simulink model "stm32f4_read_agm_imu_9a_target_demo"  (Simulink 7.3)
settings: Solver=ode3  SolverMode=SingleTasking  StartTime=0.0  StopTime=10.0  RelTol=1e-3
PreLoadFcn:
  | waijung.modelPreload; % Required for working with Waijung Blockset. Do not remove.
undefined symbols (not defined in the file): HSEOSC, Link, LQFP176, ST, STM32F417IG
libraries: simulink x21, stm32f4_i2c_lib x19, stm32f4_device_config_lib x1
CloseFcn:
  | waijung.modelClose; % Required for working with Waijung Blockset. Do not remove.
settings Model: Creator=Krisada  LastModifiedBy=Krisada
settings OptimizationCC: OptimizeModelRefInitCode=on  LifeSpan=1
settings HardwareCC: ProdEndianess=LittleEndian  ProdHWDeviceType=ARM Compatible->Cortex - M4  TargetEndianess=LittleEndian  TargetHWDeviceType=ARM Compatible->Cortex - M4
settings RTWCC: SystemTargetFile=stm32f4.tlc  GenerateMakefile=off  TemplateMakefile=ert_default_tmf  Description=STM32F4 Target  ProcessScript=stm32f4_make_rtw_hook
settings CodeAppCC: IgnoreCustomStorageClasses=off
settings STFCustomTargetCC: ModelReferenceCompliant=off  CombineOutputUpdateFcns=on  ERTCustomFileBanners=on  SupportContinuousTime=off  SupportNonInlinedSFcns=off  SystemTargetFile=stm32f4.tlc
settings ERTTargetCC: MultiwordLength=2048  ModelReferenceCompliant=off  ParMdlRefBuildCompliant=off  CompOptLevelCompliant=off  ERTFirstTimeCompliant=off  ModelStepFunctionPrototypeControlCompliant=off  CPPClassGenCompliant=off  InlinedParameterPlacement=NonHierarchical  ERTSrcFileBannerTemplate=stm32f4_code_template.cgt  ERTHdrFileBannerTemplate=stm32f4_code_template.cgt  ERTDataSrcFileTemplate=stm32f4_code_template.cgt  ERTDataHdrFileTemplate=stm32f4_code_template.cgt  ERTCustomFileTemplate=stm32f4_file_process.tlc

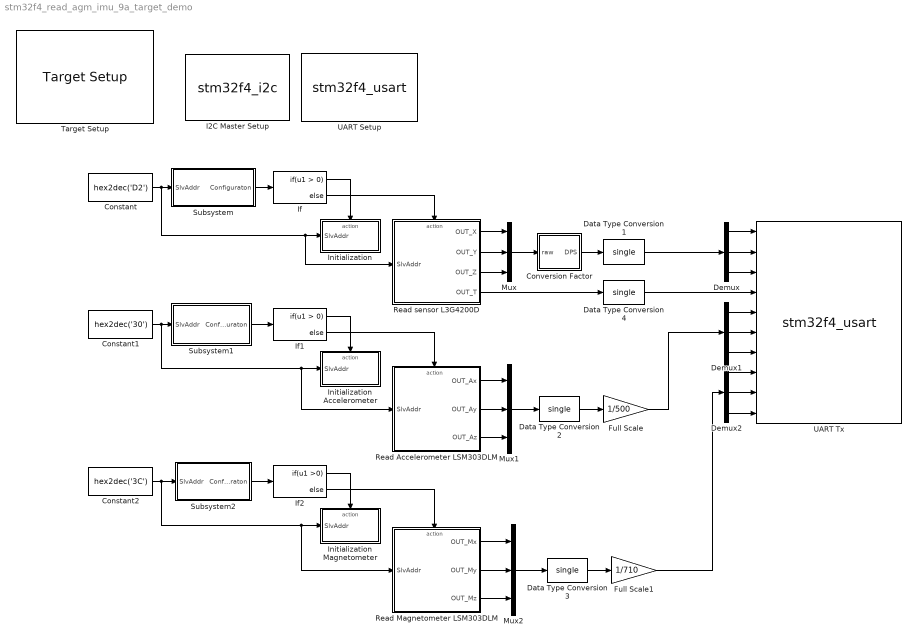
== system stm32f4_read_agm_imu_9a_target_demo ==
  Constant : Constant  Value=hex2dec('D2')  OutDataTypeMode=uint8  OutDataType=fixdt(1, 16)  OutScaling=2^0  OutDataTypeStr=uint8
  Constant1 : Constant  Value=hex2dec('30')  OutDataTypeMode=uint8  OutDataType=fixdt(1, 16)  OutScaling=2^0  OutDataTypeStr=uint8
  Constant2 : Constant  Value=hex2dec('3C')  OutDataTypeMode=uint8  OutDataType=fixdt(1, 16)  OutScaling=2^0  OutDataTypeStr=uint8
  Conversion Factor : Subsystem
  Data Type Conversion{1..4} (4 alike) : DataTypeConversion  OutDataTypeMode=single  OutDataType=fixdt(1, 16)  OutScaling=2^0  OutDataTypeStr=single
  Demux : Demux  Outputs=3
  Demux1 : Demux  Outputs=3
  Demux2 : Demux  Outputs=3
  Full Scale : Gain  Gain=1/500  ParameterDataType=fixdt(1, 16)  ParameterScaling=2^0  OutDataType=fixdt(1, 16)  OutScaling=2^0
  Full Scale1 : Gain  Gain=1/710  ParameterDataType=fixdt(1, 16)  ParameterScaling=2^0  OutDataType=fixdt(1, 16)  OutScaling=2^0
  I2C Master Setup : S-Function  FunctionName=stm32f4_i2c  Parameters=configuration,module,transfer,clkspeed,timeout,sdapin,sclpin,writecount,readcount,inputtypearray,outputtypearray,confstr,sampletime,sampletimestr,blockid  EnableBusSupport=off  mask(stm32f4_i2c){configuration=Setup, module=1, lastmodule=1, transfer=Blocking, dutycycle=TLow/THigh = 2, clkspeed=100, timeout=25, writecount=0, readcount=0, sdapin=B7, sclpin=B6, waitwritetime=0, inputtypearray=[0], outputtypearray=[0], confstr=["B","7","B","6","1","1","6","0","I2C_DutyCycle_2","0","off"], sampletime=-1, sampletimestr=0.01, blockid=I2CMasterSetup}
      mask prompts: module "I2C Module"; lastmodule "Last module"; transfer "Transfer mode"; dutycycle "Duty cycle in fast mode"; clkspeed "Clock speed (kHz)"; timeout "Timeout (ms)"; writecount "Bytes write count"; readcount "Bytes read count"; sdapin "SDA pin"; sclpin "SCL pin"; waitwritetime "Wait write time (ms), default is 0"; inputtypearray "Input type array"; outputtypearray "Output type array"; confstr "Configuration string"; sampletime "Sample time (sec)"; sampletimestr "Compiled sample time (sec) in string"
      mask init:
      | stm32f4_i2c_callback('init');
      mask Help: web(fullfile(waijungdocroot,'stm32f4_i2c_setup.htm'), '-browser')
      mask StyleString: popup(Setup|Transaction),popup(1|2|3),edit,popup(Blocking|Non-blocking),popup(TLow/THigh = 16/9|TLow/THigh = 2),edit,edit,edit,edit,popup(Not used|B7|B9),popup(Not used|B6|B8),edit,edit,edit,edit,edit,edit,edit
      mask CallbackString: stm32f4_i2c_callback('configuration');|stm32f4_i2c_callback('module');|||stm32f4_i2c_callback('dutycycle');|||stm32f4_i2c_callback('writecount');|stm32f4_i2c_callback('readcount');|stm32f4_i2c_callback('sdapin');|stm32f4_i2c_callback('sclpin');||||stm32f4_i2c_callback('confstr');|stm32f4_i2c_callback('sampletime');|stm32f4_i2c_callback('sampletimestr');|stm32f4_i2c_callback('blockid');
      mask Display: text(0.5, 0.5, 'Module: I2C1\nClock: 100kHz\nSDA/SCL Pin: B7/B6','ver','middle','hor','center');
  If : If
  If1 : If
  If2 : If  IfExpression=u1 >0
  Initialization : Subsystem
  Initialization Accelerometer : Subsystem
  Initialization Magnetometer : Subsystem
  Mux : Mux  Inputs=3
  Mux1 : Mux  Inputs=3
  Mux2 : Mux  Inputs=3
  Read Accelerometer LSM303DLM : Subsystem  TreatAsAtomicUnit=on
  Read Magnetometer LSM303DLM : Subsystem  TreatAsAtomicUnit=on
  Read sensor L3G4200D : Subsystem  TreatAsAtomicUnit=on
  Subsystem : Subsystem
  Subsystem1 : Subsystem
  Subsystem2 : Subsystem
  Target Setup : stm32f4_device_config_lib/Target Setup  Priority=100  compiler=GNU ARM  previous_compiler=GNU ARM  mcu=STM32F417IG (LQFP176)  mcustr=STM32F417IG  clockconfig=HSEOSC-8MHz  system_stm32f4xx_c_path=F:\trunk\targets\stm32f4_target\stm32f4\utils\system_stm32f4xx_default\STM32F40_41xxx\hseosc8mhz  showmemoryconfiguration=off  stacksize=0x2000  heapsize=0x2000  enableautocompiledownload=on  fullchiperase=off  programmerinterface=ST-Link  editctrlstr=on  compilercontrolstr=$(patsubst %, -I%, .) -mcpu=cortex-m4 -mthumb -mthumb-interwork -mfloat-abi=hard -mfpu=fpv4-sp-d16 -ffast-math -Wall -Wextra -Ofast  assemblercontrolstr=$(patsubst %, -I%, .) -mcpu=cortex-m4 -mthumb -mthumb-interwork -mfloat-abi=hard -mfpu=fpv4-sp-d16 -ffast-math -Wall -Wextra -Ofast -Wa,-amhls=$(<:.s=.lst) -D__STACK_SIZE=$(STACK_SIZE) -D__HEAP_SIZE=$(HEAP_SIZE)  linkercontrolstr=-T$(LD_SCRIPT) -g -Wl,-Map=$(MAP),--cref,--no-warn-mismatch -mcpu=cortex-m4 -mthumb -mthumb-interwork -mfloat-abi=hard -mfpu=fpv4-sp-d16 -specs=nosys.specs  runafterdownload=on  execprofile=None  profileruart=3  profilerbaud=500000  profilertxpin=D8  profilerinitstr=0.01,168000000,1680000,500000,0  manualsetsampletime=off  sampletime=0.01  blockid=TargetSetup  systickreloadvalue=1680000  hseval=8000000  lastprofileruart=3  hclk=168000000  flashorigin=0x8000000  flashlength=1024k  ramorigin=0x20000000  ramlength=128k  useextram=off
  UART Setup : S-Function  Priority=1  FunctionName=stm32f4_usart  Parameters=configuration,uartmodule,transfer,baudrate,inputtype,outputtype,confstr,binheaderarray,binterminatorarray,asciiheader,asciiterminator,bindatalength,packetmode,varname,sampletime,sampletimestr,blockid  EnableBusSupport=off  mask(stm32f4_usart){configuration=Setup, uartmodule=3, baudrate=115200, databits=8, parity=No, stopbit=1, remaptxpin=D8, remaprxpin=Not used, flowcontrol=None, remapctspin=Not used, remaprtspin=Not used, advanceoptions=off, rxbuffersize=512, txbuffersize=512, transfer=Blocking, packetmode=Ascii, binheader='7E 7E', binterminator='03 03', porttype_double=1, porttype_single=0, porttype_int8=1, porttype_uint8=0, porttype_int16=0, porttype_uint16=0, porttype_int32=0, porttype_uint32=0, asciiformat='%d,%f', rx_asciiterminator=CRLF (0x0D 0x0A - "\r\n"), tx_asciiterminator=CR (0x0D - "\r"), storagename=<empty>, varname=, inputtype=[0], outputtype=[0], binheaderarray=[0], binterminatorarray=[0], bindatalength=0, asciiheader='', asciiterminator=[0], sampletime=-1, sampletimestr=0.01, blockid=UARTSetup, confstr=[ "dummy", "1", "D", "8", "0", "*", "*", "0", "*", "*", "0", "*", "*", "1", "4", "3", "1", "4", "1", "512", "512", "1", "3", "115200", "8", "No", "1", "None", "USART3"], lastmodule=3}
      mask prompts: uartmodule "UART Module"; baudrate "Baud rate (bps)"; databits "Data bits"; stopbit "Stop bit"; remaptxpin "Tx Pin"; remaprxpin "Rx Pin"; flowcontrol "Hardware flow control"; remapctspin "HW Flow control, CTS Pin"; remaprtspin "HW Flow control, RTS Pin"; advanceoptions "Advance options"; rxbuffersize "Rx buffer size (bytes)"; txbuffersize "Tx buffer size (bytes)"; packetmode "Packet mode"; binheader "Binary header (example: '7E 7E')"; binterminator "Binary terminator (example: '03 03')"; porttype_double "Number of data port, type DOUBLE"; porttype_single "Number of data port, type SINGLE"; porttype_int8 "Number of data port, type INT8"; porttype_uint8 "Number of data port, type UINT8"; porttype_int16 "Number of data port, type INT16"; porttype_uint16 "Number of data port, type UINT16"; porttype_int32 "Number of data port, type INT32"; porttype_uint32 "Number of data port, type UINT32"; asciiformat "Ascii format"; rx_asciiterminator "End of packet"; tx_asciiterminator "End of packet"; storagename "Buffer"; varname "Var name"; inputtype "Input data type"; outputtype "Output data type"; binheaderarray "Binary header"; binterminatorarray "Binary terminator"; bindatalength "Binary data length"; asciiheader "Ascii header (printf format)"; asciiterminator "Ascii terminator"; sampletime "Sample time (sec)"; sampletimestr "Compiled sample time (sec) in string"; confstr "Configuration string"; lastmodule "Last module selected"
      mask help:
      | Default STM32F4DISCOVERY + aMG F4 Connect 2 + aMG USB Converter N2 settings use
      |
      | USART3, Tx D8, Rx D9 and USB Serial Converter A.
      mask init:
      | stm32f4_usart_callback('init');
      mask Help: web(fullfile(waijungdocroot,'stm32f4_usart_setup.htm'), '-browser')
      mask StyleString: popup(Setup|Tx|Rx),popup(1|2|3|4|5|6),edit,popup(8),popup(No|Odd|Even),popup(0.5|1|1.5|2),popup(Not used|B10|C10|D8),popup(Not used|B11|C11|D9),popup(None|RTS|CTS|RTS/CTS),popup(Not used|B13|D11),popup(Not used|B14|D12),checkbox,popup(16|32|64|128|256|512|1024|2048),popup(16|32|64|128|256|512|1024|2048),popup(Blocking|Non-Blocking),popup(Ascii|Binary|String Buffer),edit,edit,edit,edit,edit,edit,edit,edit,edit,edit,edit,popup(CR (0x0D - "\r")|LF (0x0A - "\n")|CRLF (0x0D 0x0A - "\r\n")),popup(CR (0x0D - "\r")|LF (0x0A - "\n")|CRLF (0x0D 0x0A - "\r\n")|None),popup(<empty>),edit,edit,edit,edit,edit,edit,edit,edit,edit,edit,edit,edit,edit
      mask CallbackString: stm32f4_usart_callback('configuration');|stm32f4_usart_callback('uartmodule');|stm32f4_usart_callback('baudrate');||||||stm32f4_usart_callback('flowcontrol');|||stm32f4_usart_callback('advanceoptions');|||stm32f4_usart_callback('transfer');|stm32f4_usart_callback('packetmode');|stm32f4_usart_callback('binheader');|stm32f4_usart_callback('binterminator');|stm32f4_usart_callback('porttype');|stm32f4_usart_callback('porttype');|stm32f4_usart_callback('porttype');|stm32f4_usart_callback('porttype');|stm32f4_usart_callback('porttype');|stm32f4_usart_callback('porttype');|stm32f4_usart_callback('porttype');|stm32f4_usart_callback('porttype');|stm32f4_usart_callback('asciiformat');|stm32f4_usart_callback('rx_asciiterminator');|stm32f4_usart_callback('tx_asciiterminator');|stm32f4_usart_callback('storagename');|stm32f4_usart_callback('varname');||||||||stm32f4_usart_callback('sampletime');|stm32f4_usart_callback('sampletimestr');|stm32f4_usart_callback('blockid');||
      mask Display: text(0.5, 0.5, 'Module: USART3_Setup\nBaud (Bps): 115200\nDMA Buffer: 512/-\nTx/Rx Pin: D8/-','ver','middle','hor','center');
  UART Tx : S-Function  Priority=1  FunctionName=stm32f4_usart  Parameters=configuration,uartmodule,transfer,baudrate,inputtype,outputtype,confstr,binheaderarray,binterminatorarray,asciiheader,asciiterminator,bindatalength,packetmode,varname,sampletime,sampletimestr,blockid  EnableBusSupport=off  mask(stm32f4_usart){configuration=Tx, uartmodule=3, baudrate=115200, databits=8, parity=No, stopbit=1, remaptxpin=Not used, remaprxpin=Not used, flowcontrol=None, remapctspin=Not used, remaprtspin=Not used, advanceoptions=off, rxbuffersize=512, txbuffersize=512, transfer=Blocking, packetmode=Binary, binheader='7E 7E', binterminator='03 03', porttype_double=0, porttype_single=10, porttype_int8=0, porttype_uint8=0, porttype_int16=0, porttype_uint16=0, porttype_int32=0, porttype_uint32=0, asciiformat='value=%d,%f', rx_asciiterminator=CRLF (0x0D 0x0A - "\r\n"), tx_asciiterminator=CRLF (0x0D 0x0A - "\r\n"), storagename=<empty>, varname=, inputtype=[10  1 1 1 1 1 1 1 1 1 1], outputtype=[0], binheaderarray=[2 126  126], binterminatorarray=[2 3  3], bindatalength=40, asciiheader='value=%d,%f\r\n', asciiterminator=[2 13 10], sampletime=-1, sampletimestr=0.01, blockid=UARTTx, confstr=[ "dummy", "0", "*", "*", "0", "*", "*", "0", "*", "*", "0", "*", "*", "1", "4", "3", "1", "4", "1", "512", "512", "1", "3", "115200", "8", "No", "1", "None", "USART3"], lastmodule=1}
      mask prompts: uartmodule "UART Module"; baudrate "Baud rate (bps)"; databits "Data bits"; stopbit "Stop bit"; remaptxpin "Tx Pin"; remaprxpin "Rx Pin"; flowcontrol "Hardware flow control"; remapctspin "HW Flow control, CTS Pin"; remaprtspin "HW Flow control, RTS Pin"; advanceoptions "Advance options"; rxbuffersize "Rx buffer size (bytes)"; txbuffersize "Tx buffer size (bytes)"; packetmode "Packet mode"; binheader "Binary header (example: '7E 7E')"; binterminator "Binary terminator (example: '03 03')"; porttype_double "Number of data port, type DOUBLE"; porttype_single "Number of data port, type SINGLE"; porttype_int8 "Number of data port, type INT8"; porttype_uint8 "Number of data port, type UINT8"; porttype_int16 "Number of data port, type INT16"; porttype_uint16 "Number of data port, type UINT16"; porttype_int32 "Number of data port, type INT32"; porttype_uint32 "Number of data port, type UINT32"; asciiformat "Ascii format"; rx_asciiterminator "End of packet"; tx_asciiterminator "End of packet"; storagename "Buffer"; varname "Var name"; inputtype "Input data type"; outputtype "Output data type"; binheaderarray "Binary header"; binterminatorarray "Binary terminator"; bindatalength "Binary data length"; asciiheader "Ascii header (printf format)"; asciiterminator "Ascii terminator"; sampletime "Sample time (sec)"; sampletimestr "Compiled sample time (sec) in string"; confstr "Configuration string"; lastmodule "Last module selected"
      mask help:
      | Data type for Ascii format
      | %u, %i, %d, %o, %x: uint32
      | %e, %g, %f: single
      | %c: int8
      mask init:
      | stm32f4_usart_callback('init');
      mask Help: web(fullfile(waijungdocroot,'stm32f4_usart_tx.htm'), '-browser')
      mask StyleString: popup(Setup|Tx|Rx),popup(1|2|3|4|5|6),edit,popup(8),popup(No|Odd|Even),popup(0.5|1|1.5|2),popup(Not used|A9|B6),popup(Not used|A10|B7),popup(None|RTS|CTS|RTS/CTS),popup(Not used|A11),popup(Not used|A12),checkbox,popup(16|32|64|128|256|512|1024|2048),popup(16|32|64|128|256|512|1024|2048),popup(Blocking|Non-Blocking),popup(Ascii|Binary|String Buffer),edit,edit,edit,edit,edit,edit,edit,edit,edit,edit,edit,popup(CR (0x0D - "\r")|LF (0x0A - "\n")|CRLF (0x0D 0x0A - "\r\n")),popup(CR (0x0D - "\r")|LF (0x0A - "\n")|CRLF (0x0D 0x0A - "\r\n")|None),popup(<empty>),edit,edit,edit,edit,edit,edit,edit,edit,edit,edit,edit,edit,edit
      mask CallbackString: stm32f4_usart_callback('configuration');|stm32f4_usart_callback('uartmodule');|stm32f4_usart_callback('baudrate');||||||stm32f4_usart_callback('flowcontrol');|||stm32f4_usart_callback('advanceoptions');|||stm32f4_usart_callback('transfer');|stm32f4_usart_callback('packetmode');|stm32f4_usart_callback('binheader');|stm32f4_usart_callback('binterminator');|stm32f4_usart_callback('porttype');|stm32f4_usart_callback('porttype');|stm32f4_usart_callback('porttype');|stm32f4_usart_callback('porttype');|stm32f4_usart_callback('porttype');|stm32f4_usart_callback('porttype');|stm32f4_usart_callback('porttype');|stm32f4_usart_callback('porttype');|stm32f4_usart_callback('asciiformat');|stm32f4_usart_callback('rx_asciiterminator');|stm32f4_usart_callback('tx_asciiterminator');|stm32f4_usart_callback('storagename');|stm32f4_usart_callback('varname');||||||||stm32f4_usart_callback('sampletime');|stm32f4_usart_callback('sampletimestr');|stm32f4_usart_callback('blockid');||
      mask Display: text(0.95, 0.5, 'Module: USART3_Tx\nPacket: Binary\nTransfer: Blocking\nTs (sec): 0.01','ver','middle','hor','right'); port_label('input', 1,'single'); port_label('input', 2,'single'); port_label('input', 3,'single'); port_label('input', 4,'single'); port_label('input', 5,'single'); port_label('input', 6,'single'); port_label('input', 7,'single'); port_label('input', 8,'single'); port_label('input', 9,'single'); port_label('input', 10,'single');
  wires:
  Subsystem/1(Configuraton) -> If/1
  Read sensor L3G4200D/1(OUT_X) -> Mux/1
  Read sensor L3G4200D/2(OUT_Y) -> Mux/2
  Read sensor L3G4200D/3(OUT_Z) -> Mux/3
  Conversion Factor/1(DPS) -> Data Type Conversion1/1
  Mux/1 -> Conversion Factor/1(raw)
  Data Type Conversion1/1 -> Demux/1
  If/1 -> Initialization/Action
  If/2 -> Read sensor L3G4200D/Action
  Subsystem1/1(Configuraton) -> If1/1
  Read Accelerometer LSM303DLM/1(OUT_Ax) -> Mux1/1
  Data Type Conversion2/1 -> Full Scale/1
  If1/1 -> Initialization Accelerometer/Action
  If1/2 -> Read Accelerometer LSM303DLM/Action
  Read Accelerometer LSM303DLM/2(OUT_Ay) -> Mux1/2
  Read Accelerometer LSM303DLM/3(OUT_Az) -> Mux1/3
  Mux1/1 -> Data Type Conversion2/1
  Full Scale/1 -> Demux1/1
  Read Magnetometer LSM303DLM/1(OUT_Mx) -> Mux2/1
  Data Type Conversion3/1 -> Full Scale1/1
  If2/1 -> Initialization Magnetometer/Action
  If2/2 -> Read Magnetometer LSM303DLM/Action
  Read Magnetometer LSM303DLM/2(OUT_My) -> Mux2/2
  Read Magnetometer LSM303DLM/3(OUT_Mz) -> Mux2/3
  Mux2/1 -> Data Type Conversion3/1
  Full Scale1/1 -> Demux2/1
  Subsystem2/1(Configuraton) -> If2/1
  Constant/1 -> Subsystem/1(SlvAddr), Initialization/1(SlvAddr), Read sensor L3G4200D/1(SlvAddr)
  Constant1/1 -> Subsystem1/1(SlvAddr), Initialization Accelerometer/1(SlvAddr), Read Accelerometer LSM303DLM/1(SlvAddr)
  Constant2/1 -> Subsystem2/1(SlvAddr), Initialization Magnetometer/1(SlvAddr), Read Magnetometer LSM303DLM/1(SlvAddr)
  Read sensor L3G4200D/4(OUT_T) -> Data Type Conversion4/1
  Demux/1 -> UART Tx/1
  Demux/2 -> UART Tx/2
  Demux/3 -> UART Tx/3
  Demux1/1 -> UART Tx/5
  Demux1/2 -> UART Tx/6
  Demux1/3 -> UART Tx/7
  Demux2/1 -> UART Tx/8
  Demux2/2 -> UART Tx/9
  Demux2/3 -> UART Tx/10
  Data Type Conversion4/1 -> UART Tx/4

== system stm32f4_read_agm_imu_9a_target_demo/Conversion Factor ==
  raw : Inport
  Constant : Constant  Value=2^15  OutDataType=fixdt(1, 16)  OutScaling=2^0
  Divide : Product  Inputs=*/  OutDataType=fixdt(1, 16)  OutScaling=2^-10
  Full Scale : Gain  Gain=250  ParameterDataType=fixdt(1, 16)  ParameterScaling=2^0  OutDataType=fixdt(1, 16)  OutScaling=2^0
  DPS : Outport
  wires:
  Constant/1 -> Divide/2
  Divide/1 -> Full Scale/1
  raw/1 -> Divide/1
  Full Scale/1 -> DPS/1

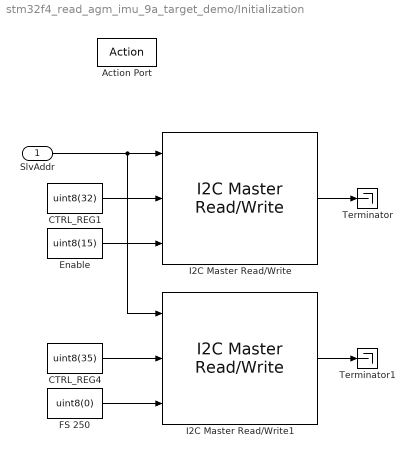
== system stm32f4_read_agm_imu_9a_target_demo/Initialization ==
  SlvAddr : Inport  OutDataType=fixdt(1, 16)  OutScaling=2^0
  Action Port : ActionPort  ActionType=then
  CTRL_REG1 : Constant  Value=uint8(32)  OutDataType=fixdt(1, 16)  OutScaling=2^0
  CTRL_REG4 : Constant  Value=uint8(35)  OutDataType=fixdt(1, 16)  OutScaling=2^0
  Enable : Constant  Value=uint8(15)  OutDataType=fixdt(1, 16)  OutScaling=2^0
  FS 250 : Constant  Value=uint8(0)  OutDataType=fixdt(1, 16)  OutScaling=2^0
  I2C Master Read/Write : stm32f4_i2c_lib/I2C Master Read//Write  configuration=Transaction  module=1  lastmodule=3  transfer=Blocking  dutycycle=TLow/THigh = 2  clkspeed=400  timeout=25  writecount=2  readcount=0  sdapin=C9  sclpin=A8  waitwritetime=0  forcestop=off  inputtypearray=[3 3 3 3]  outputtypearray=[1 3]  confstr="[\"C\",\"9\",\"A\",\"8\",\"1\",\"1\",\"6\",\"0\",\"I2C_DutyCycle_2\",\"0\",\"off\"]"  sampletime=-1  sampletimestr=0.01  blockid=InitializationI2CMasterReadWrite
  I2C Master Read/Write1 : stm32f4_i2c_lib/I2C Master Read//Write  configuration=Transaction  module=1  lastmodule=3  transfer=Blocking  dutycycle=TLow/THigh = 2  clkspeed=400  timeout=25  writecount=2  readcount=0  sdapin=C9  sclpin=A8  waitwritetime=0  forcestop=off  inputtypearray=[3 3 3 3]  outputtypearray=[1 3]  confstr="[\"C\",\"9\",\"A\",\"8\",\"1\",\"1\",\"6\",\"0\",\"I2C_DutyCycle_2\",\"0\",\"off\"]"  sampletime=-1  sampletimestr=0.01  blockid=InitializationI2CMasterReadWrite1
  Terminator : Terminator
  Terminator1 : Terminator
  wires:
  CTRL_REG1/1 -> I2C Master Read/Write/2
  Enable/1 -> I2C Master Read/Write/3
  CTRL_REG4/1 -> I2C Master Read/Write1/2
  FS 250/1 -> I2C Master Read/Write1/3
  SlvAddr/1 -> I2C Master Read/Write/1, I2C Master Read/Write1/1
  I2C Master Read/Write/1 -> Terminator/1
  I2C Master Read/Write1/1 -> Terminator1/1

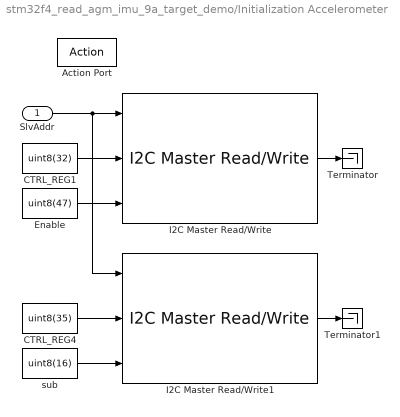
== system stm32f4_read_agm_imu_9a_target_demo/Initialization Accelerometer ==
  SlvAddr : Inport  OutDataType=fixdt(1, 16)  OutScaling=2^0
  Action Port : ActionPort  ActionType=then
  CTRL_REG1 : Constant  Value=uint8(32)  OutDataType=fixdt(1, 16)  OutScaling=2^0
  CTRL_REG4 : Constant  Value=uint8(35)  OutDataType=fixdt(1, 16)  OutScaling=2^0
  Enable : Constant  Value=uint8(47)  OutDataType=fixdt(1, 16)  OutScaling=2^0
  I2C Master Read/Write : stm32f4_i2c_lib/I2C Master Read//Write  configuration=Transaction  module=1  lastmodule=3  transfer=Blocking  dutycycle=TLow/THigh = 2  clkspeed=400  timeout=25  writecount=2  readcount=0  sdapin=C9  sclpin=A8  waitwritetime=0  forcestop=off  inputtypearray=[3 3 3 3]  outputtypearray=[1 3]  confstr="[\"C\",\"9\",\"A\",\"8\",\"1\",\"1\",\"6\",\"0\",\"I2C_DutyCycle_2\",\"0\",\"off\"]"  sampletime=-1  sampletimestr=0.01  blockid=InitializationAccelerometerI2CMasterReadWrite
  I2C Master Read/Write1 : stm32f4_i2c_lib/I2C Master Read//Write  configuration=Transaction  module=1  lastmodule=3  transfer=Blocking  dutycycle=TLow/THigh = 2  clkspeed=400  timeout=25  writecount=2  readcount=0  sdapin=C9  sclpin=A8  waitwritetime=0  forcestop=off  inputtypearray=[3 3 3 3]  outputtypearray=[1 3]  confstr="[\"C\",\"9\",\"A\",\"8\",\"1\",\"1\",\"6\",\"0\",\"I2C_DutyCycle_2\",\"0\",\"off\"]"  sampletime=-1  sampletimestr=0.01  blockid=InitializationAccelerometerI2CMasterReadWrite1
  Terminator : Terminator
  Terminator1 : Terminator
  sub : Constant  Value=uint8(16)  OutDataType=fixdt(1, 16)  OutScaling=2^0
  wires:
  Enable/1 -> I2C Master Read/Write/3
  CTRL_REG1/1 -> I2C Master Read/Write/2
  sub/1 -> I2C Master Read/Write1/3
  CTRL_REG4/1 -> I2C Master Read/Write1/2
  SlvAddr/1 -> I2C Master Read/Write/1, I2C Master Read/Write1/1
  I2C Master Read/Write/1 -> Terminator/1
  I2C Master Read/Write1/1 -> Terminator1/1

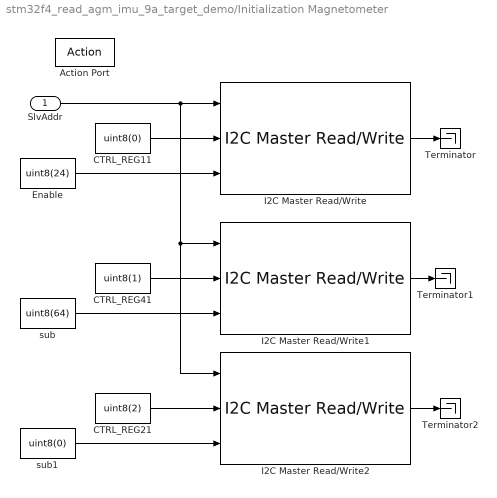
== system stm32f4_read_agm_imu_9a_target_demo/Initialization Magnetometer ==
  SlvAddr : Inport  OutDataType=fixdt(1, 16)  OutScaling=2^0
  Action Port : ActionPort  ActionType=then
  CTRL_REG11 : Constant  Value=uint8(0)  OutDataType=fixdt(1, 16)  OutScaling=2^0
  CTRL_REG21 : Constant  Value=uint8(2)  OutDataType=fixdt(1, 16)  OutScaling=2^0
  CTRL_REG41 : Constant  Value=uint8(1)  OutDataType=fixdt(1, 16)  OutScaling=2^0
  Enable : Constant  Value=uint8(24)  OutDataType=fixdt(1, 16)  OutScaling=2^0
  I2C Master Read/Write : stm32f4_i2c_lib/I2C Master Read//Write  configuration=Transaction  module=1  lastmodule=3  transfer=Blocking  dutycycle=TLow/THigh = 2  clkspeed=400  timeout=25  writecount=2  readcount=0  sdapin=C9  sclpin=A8  waitwritetime=0  forcestop=off  inputtypearray=[3 3 3 3]  outputtypearray=[1 3]  confstr="[\"C\",\"9\",\"A\",\"8\",\"1\",\"1\",\"6\",\"0\",\"I2C_DutyCycle_2\",\"0\",\"off\"]"  sampletime=-1  sampletimestr=0.01  blockid=InitializationMagnetometerI2CMasterReadWrite
  I2C Master Read/Write1 : stm32f4_i2c_lib/I2C Master Read//Write  configuration=Transaction  module=1  lastmodule=3  transfer=Blocking  dutycycle=TLow/THigh = 2  clkspeed=400  timeout=25  writecount=2  readcount=0  sdapin=C9  sclpin=A8  waitwritetime=0  forcestop=off  inputtypearray=[3 3 3 3]  outputtypearray=[1 3]  confstr="[\"C\",\"9\",\"A\",\"8\",\"1\",\"1\",\"6\",\"0\",\"I2C_DutyCycle_2\",\"0\",\"off\"]"  sampletime=-1  sampletimestr=0.01  blockid=InitializationMagnetometerI2CMasterReadWrite1
  I2C Master Read/Write2 : stm32f4_i2c_lib/I2C Master Read//Write  configuration=Transaction  module=1  lastmodule=3  transfer=Blocking  dutycycle=TLow/THigh = 2  clkspeed=400  timeout=25  writecount=2  readcount=0  sdapin=C9  sclpin=A8  waitwritetime=0  forcestop=off  inputtypearray=[3 3 3 3]  outputtypearray=[1 3]  confstr="[\"C\",\"9\",\"A\",\"8\",\"1\",\"1\",\"6\",\"0\",\"I2C_DutyCycle_2\",\"0\",\"off\"]"  sampletime=-1  sampletimestr=0.01  blockid=InitializationMagnetometerI2CMasterReadWrite2
  Terminator : Terminator
  Terminator1 : Terminator
  Terminator2 : Terminator
  sub : Constant  Value=uint8(64)  OutDataType=fixdt(1, 16)  OutScaling=2^0
  sub1 : Constant  Value=uint8(0)  OutDataType=fixdt(1, 16)  OutScaling=2^0
  wires:
  CTRL_REG11/1 -> I2C Master Read/Write/2
  Enable/1 -> I2C Master Read/Write/3
  CTRL_REG41/1 -> I2C Master Read/Write1/2
  sub/1 -> I2C Master Read/Write1/3
  I2C Master Read/Write/1 -> Terminator/1
  SlvAddr/1 -> I2C Master Read/Write/1, I2C Master Read/Write1/1, I2C Master Read/Write2/1
  sub1/1 -> I2C Master Read/Write2/3
  CTRL_REG21/1 -> I2C Master Read/Write2/2
  I2C Master Read/Write1/1 -> Terminator1/1
  I2C Master Read/Write2/1 -> Terminator2/1

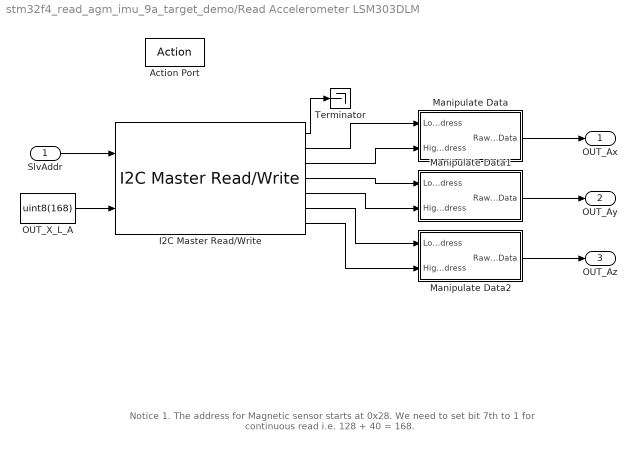
== system stm32f4_read_agm_imu_9a_target_demo/Read Accelerometer LSM303DLM ==
  note: Notice
      | 1. The address for Magnetic sensor starts at 0x28. We need to set bit 7th to 1 for continuous read i.e. 128 + 40 = 168.
  SlvAddr : Inport  OutDataType=fixdt(1, 16)  OutScaling=2^0
  Action Port : ActionPort  ActionType=else
  I2C Master Read/Write : stm32f4_i2c_lib/I2C Master Read//Write  configuration=Transaction  module=1  lastmodule=3  transfer=Blocking  dutycycle=TLow/THigh = 2  clkspeed=400  timeout=25  writecount=1  readcount=6  sdapin=C9  sclpin=A8  waitwritetime=0  forcestop=off  inputtypearray=[2 3 3]  outputtypearray=[7 3 3 3 3 3 3 3]  confstr="[\"C\",\"9\",\"A\",\"8\",\"1\",\"1\",\"6\",\"0\",\"I2C_DutyCycle_2\",\"0\",\"off\"]"  sampletime=-1  sampletimestr=0.01  blockid=ReadAccelerometerLSM303DLMI2CMasterReadWrite
  Manipulate Data : Subsystem
  Manipulate Data1 : Subsystem
  Manipulate Data2 : Subsystem
  OUT_X_L_A : Constant  Value=uint8(168)  OutDataType=fixdt(1, 16)  OutScaling=2^0
  Terminator : Terminator
  OUT_Ax : Outport  OutDataType=fixdt(1, 16)  OutScaling=2^0
  OUT_Ay : Outport  Port=2  OutDataType=fixdt(1, 16)  OutScaling=2^0
  OUT_Az : Outport  Port=3  OutDataType=fixdt(1, 16)  OutScaling=2^0
  wires:
  OUT_X_L_A/1 -> I2C Master Read/Write/2
  Manipulate Data/1(RawAccData) -> OUT_Ax/1
  Manipulate Data1/1(RawAccData) -> OUT_Ay/1
  Manipulate Data2/1(RawAccData) -> OUT_Az/1
  I2C Master Read/Write/1 -> Terminator/1
  I2C Master Read/Write/2 -> Manipulate Data/1(LowAddress)
  I2C Master Read/Write/3 -> Manipulate Data/2(HighAddress)
  I2C Master Read/Write/4 -> Manipulate Data1/1(LowAddress)
  I2C Master Read/Write/5 -> Manipulate Data1/2(HighAddress)
  I2C Master Read/Write/6 -> Manipulate Data2/1(LowAddress)
  I2C Master Read/Write/7 -> Manipulate Data2/2(HighAddress)
  SlvAddr/1 -> I2C Master Read/Write/1

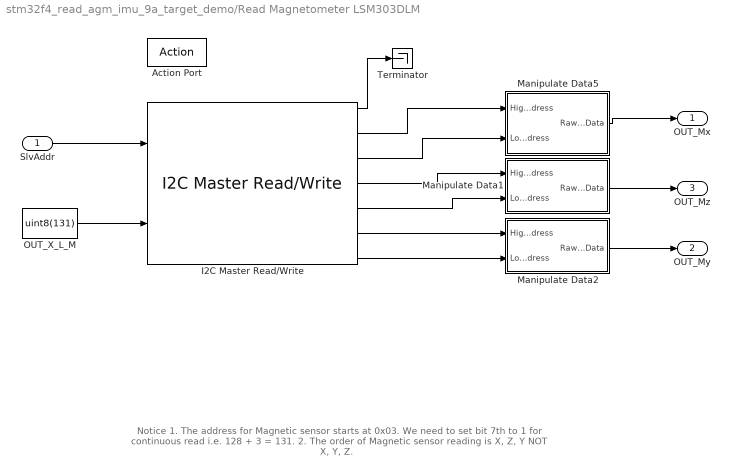
== system stm32f4_read_agm_imu_9a_target_demo/Read Magnetometer LSM303DLM ==
  note: Notice
      | 1. The address for Magnetic sensor starts at 0x03. We need to set bit 7th to 1 for continuous read i.e. 128 + 3 = 131.
      | 2. The order of Magnetic sensor reading is X, Z, Y NOT X, Y, Z.
  SlvAddr : Inport  OutDataType=fixdt(1, 16)  OutScaling=2^0
  Action Port : ActionPort  ActionType=else
  I2C Master Read/Write : stm32f4_i2c_lib/I2C Master Read//Write  configuration=Transaction  module=1  lastmodule=3  transfer=Blocking  dutycycle=TLow/THigh = 2  clkspeed=400  timeout=25  writecount=1  readcount=6  sdapin=C9  sclpin=A8  waitwritetime=0  forcestop=off  inputtypearray=[2 3 3]  outputtypearray=[7 3 3 3 3 3 3 3]  confstr="[\"C\",\"9\",\"A\",\"8\",\"1\",\"1\",\"6\",\"0\",\"I2C_DutyCycle_2\",\"0\",\"off\"]"  sampletime=-1  sampletimestr=0.01  blockid=ReadMagnetometerLSM303DLMI2CMasterReadWrite
  Manipulate Data1 : Subsystem
  Manipulate Data2 : Subsystem
  Manipulate Data5 : Subsystem
  OUT_X_L_M : Constant  Value=uint8(131)  OutDataType=fixdt(1, 16)  OutScaling=2^0
  Terminator : Terminator
  OUT_Mx : Outport  OutDataType=fixdt(1, 16)  OutScaling=2^0
  OUT_My : Outport  Port=2  OutDataType=fixdt(1, 16)  OutScaling=2^0
  OUT_Mz : Outport  Port=3  OutDataType=fixdt(1, 16)  OutScaling=2^0
  wires:
  Manipulate Data5/1(RawMagData) -> OUT_Mx/1
  OUT_X_L_M/1 -> I2C Master Read/Write/2
  Manipulate Data1/1(RawMagData) -> OUT_Mz/1
  Manipulate Data2/1(RawMagData) -> OUT_My/1
  SlvAddr/1 -> I2C Master Read/Write/1
  I2C Master Read/Write/1 -> Terminator/1
  I2C Master Read/Write/2 -> Manipulate Data5/1(HighAddress)
  I2C Master Read/Write/3 -> Manipulate Data5/2(LowAddress)
  I2C Master Read/Write/4 -> Manipulate Data1/1(HighAddress)
  I2C Master Read/Write/5 -> Manipulate Data1/2(LowAddress)
  I2C Master Read/Write/6 -> Manipulate Data2/1(HighAddress)
  I2C Master Read/Write/7 -> Manipulate Data2/2(LowAddress)

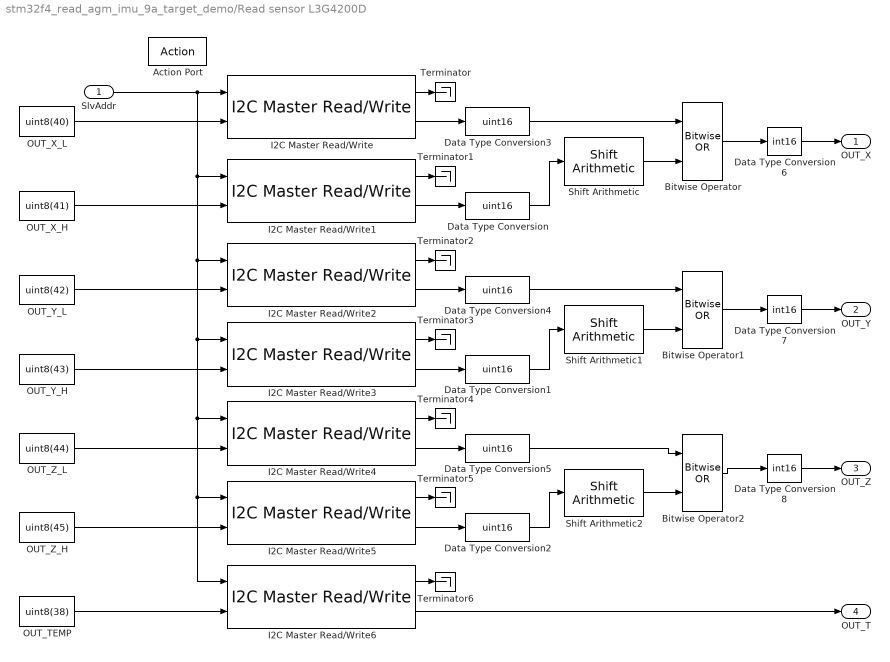
== system stm32f4_read_agm_imu_9a_target_demo/Read sensor L3G4200D ==
  SlvAddr : Inport  OutDataType=fixdt(1, 16)  OutScaling=2^0
  Action Port : ActionPort  ActionType=else
  Bitwise Operator : simulink/Logic and Bit Operations/Bitwise Operator  logicop=OR  UseBitMask=off  NumInputPorts=2  BitMask=bin2dec('11011001')  BitMaskRealWorld=Stored Integer
  Bitwise Operator1 : simulink/Logic and Bit Operations/Bitwise Operator  logicop=OR  UseBitMask=off  NumInputPorts=2  BitMask=bin2dec('11011001')  BitMaskRealWorld=Stored Integer
  Bitwise Operator2 : simulink/Logic and Bit Operations/Bitwise Operator  logicop=OR  UseBitMask=off  NumInputPorts=2  BitMask=bin2dec('11011001')  BitMaskRealWorld=Stored Integer
  Data Type Conversion{,1..5} (6 alike) : DataTypeConversion  OutDataTypeMode=uint16  OutDataType=fixdt(1, 16)  OutScaling=2^0  OutDataTypeStr=uint16
  Data Type Conversion6 : DataTypeConversion  OutDataTypeMode=int16  OutDataType=fixdt(1, 16)  OutScaling=2^0  OutDataTypeStr=int16
  Data Type Conversion7 : DataTypeConversion  OutDataTypeMode=int16  OutDataType=fixdt(1, 16)  OutScaling=2^0  OutDataTypeStr=int16
  Data Type Conversion8 : DataTypeConversion  OutDataTypeMode=int16  OutDataType=fixdt(1, 16)  OutScaling=2^0  OutDataTypeStr=int16
  I2C Master Read/Write : stm32f4_i2c_lib/I2C Master Read//Write  configuration=Transaction  module=1  lastmodule=3  transfer=Blocking  dutycycle=TLow/THigh = 2  clkspeed=400  timeout=25  writecount=1  readcount=1  sdapin=C9  sclpin=A8  waitwritetime=0  forcestop=off  inputtypearray=[2 3 3]  outputtypearray=[2 3 3]  confstr="[\"C\",\"9\",\"A\",\"8\",\"1\",\"1\",\"6\",\"0\",\"I2C_DutyCycle_2\",\"0\",\"off\"]"  sampletime=-1  sampletimestr=0.01  blockid=ReadsensorL3G4200DI2CMasterReadWrite
  I2C Master Read/Write1 : stm32f4_i2c_lib/I2C Master Read//Write  configuration=Transaction  module=1  lastmodule=3  transfer=Blocking  dutycycle=TLow/THigh = 2  clkspeed=400  timeout=25  writecount=1  readcount=1  sdapin=C9  sclpin=A8  waitwritetime=0  forcestop=off  inputtypearray=[2 3 3]  outputtypearray=[2 3 3]  confstr="[\"C\",\"9\",\"A\",\"8\",\"1\",\"1\",\"6\",\"0\",\"I2C_DutyCycle_2\",\"0\",\"off\"]"  sampletime=-1  sampletimestr=0.01  blockid=ReadsensorL3G4200DI2CMasterReadWrite1
  I2C Master Read/Write2 : stm32f4_i2c_lib/I2C Master Read//Write  configuration=Transaction  module=1  lastmodule=3  transfer=Blocking  dutycycle=TLow/THigh = 2  clkspeed=400  timeout=25  writecount=1  readcount=1  sdapin=C9  sclpin=A8  waitwritetime=0  forcestop=off  inputtypearray=[2 3 3]  outputtypearray=[2 3 3]  confstr="[\"C\",\"9\",\"A\",\"8\",\"1\",\"1\",\"6\",\"0\",\"I2C_DutyCycle_2\",\"0\",\"off\"]"  sampletime=-1  sampletimestr=0.01  blockid=ReadsensorL3G4200DI2CMasterReadWrite2
  I2C Master Read/Write3 : stm32f4_i2c_lib/I2C Master Read//Write  configuration=Transaction  module=1  lastmodule=3  transfer=Blocking  dutycycle=TLow/THigh = 2  clkspeed=400  timeout=25  writecount=1  readcount=1  sdapin=C9  sclpin=A8  waitwritetime=0  forcestop=off  inputtypearray=[2 3 3]  outputtypearray=[2 3 3]  confstr="[\"C\",\"9\",\"A\",\"8\",\"1\",\"1\",\"6\",\"0\",\"I2C_DutyCycle_2\",\"0\",\"off\"]"  sampletime=-1  sampletimestr=0.01  blockid=ReadsensorL3G4200DI2CMasterReadWrite3
  I2C Master Read/Write4 : stm32f4_i2c_lib/I2C Master Read//Write  configuration=Transaction  module=1  lastmodule=3  transfer=Blocking  dutycycle=TLow/THigh = 2  clkspeed=400  timeout=25  writecount=1  readcount=1  sdapin=C9  sclpin=A8  waitwritetime=0  forcestop=off  inputtypearray=[2 3 3]  outputtypearray=[2 3 3]  confstr="[\"C\",\"9\",\"A\",\"8\",\"1\",\"1\",\"6\",\"0\",\"I2C_DutyCycle_2\",\"0\",\"off\"]"  sampletime=-1  sampletimestr=0.01  blockid=ReadsensorL3G4200DI2CMasterReadWrite4
  I2C Master Read/Write5 : stm32f4_i2c_lib/I2C Master Read//Write  configuration=Transaction  module=1  lastmodule=3  transfer=Blocking  dutycycle=TLow/THigh = 2  clkspeed=400  timeout=25  writecount=1  readcount=1  sdapin=C9  sclpin=A8  waitwritetime=0  forcestop=off  inputtypearray=[2 3 3]  outputtypearray=[2 3 3]  confstr="[\"C\",\"9\",\"A\",\"8\",\"1\",\"1\",\"6\",\"0\",\"I2C_DutyCycle_2\",\"0\",\"off\"]"  sampletime=-1  sampletimestr=0.01  blockid=ReadsensorL3G4200DI2CMasterReadWrite5
  I2C Master Read/Write6 : stm32f4_i2c_lib/I2C Master Read//Write  configuration=Transaction  module=1  lastmodule=3  transfer=Blocking  dutycycle=TLow/THigh = 2  clkspeed=400  timeout=25  writecount=1  readcount=1  sdapin=C9  sclpin=A8  waitwritetime=0  forcestop=off  inputtypearray=[2 3 3]  outputtypearray=[2 3 3]  confstr="[\"C\",\"9\",\"A\",\"8\",\"1\",\"1\",\"6\",\"0\",\"I2C_DutyCycle_2\",\"0\",\"off\"]"  sampletime=-1  sampletimestr=0.01  blockid=ReadsensorL3G4200DI2CMasterReadWrite6
  OUT_TEMP : Constant  Value=uint8(38)  OutDataType=fixdt(1, 16)  OutScaling=2^0
  OUT_X_H : Constant  Value=uint8(41)  OutDataType=fixdt(1, 16)  OutScaling=2^0
  OUT_X_L : Constant  Value=uint8(40)  OutDataType=fixdt(1, 16)  OutScaling=2^0
  OUT_Y_H : Constant  Value=uint8(43)  OutDataType=fixdt(1, 16)  OutScaling=2^0
  OUT_Y_L : Constant  Value=uint8(42)  OutDataType=fixdt(1, 16)  OutScaling=2^0
  OUT_Z_H : Constant  Value=uint8(45)  OutDataType=fixdt(1, 16)  OutScaling=2^0
  OUT_Z_L : Constant  Value=uint8(44)  OutDataType=fixdt(1, 16)  OutScaling=2^0
  Shift Arithmetic : simulink/Logic and Bit Operations/Shift Arithmetic  SystemSampleTime=-1  nBitShiftRight=-8  nBinPtShiftRight=0
  Shift Arithmetic1 : simulink/Logic and Bit Operations/Shift Arithmetic  SystemSampleTime=-1  nBitShiftRight=-8  nBinPtShiftRight=0
  Shift Arithmetic2 : simulink/Logic and Bit Operations/Shift Arithmetic  SystemSampleTime=-1  nBitShiftRight=-8  nBinPtShiftRight=0
  Terminator{,1..6} (7 alike) : Terminator
  OUT_X : Outport  OutDataType=fixdt(1, 16)  OutScaling=2^0
  OUT_Y : Outport  Port=2  OutDataType=fixdt(1, 16)  OutScaling=2^0
  OUT_Z : Outport  Port=3  OutDataType=fixdt(1, 16)  OutScaling=2^0
  OUT_T : Outport  Port=4  OutDataType=fixdt(1, 16)  OutScaling=2^0
  wires:
  OUT_X_L/1 -> I2C Master Read/Write/2
  OUT_X_H/1 -> I2C Master Read/Write1/2
  I2C Master Read/Write1/2 -> Data Type Conversion/1
  Data Type Conversion/1 -> Shift Arithmetic/1
  I2C Master Read/Write/2 -> Data Type Conversion3/1
  Shift Arithmetic/1 -> Bitwise Operator/2
  Bitwise Operator/1 -> Data Type Conversion6/1
  OUT_Y_L/1 -> I2C Master Read/Write2/2
  OUT_Y_H/1 -> I2C Master Read/Write3/2
  I2C Master Read/Write3/2 -> Data Type Conversion1/1
  Data Type Conversion1/1 -> Shift Arithmetic1/1
  I2C Master Read/Write2/2 -> Data Type Conversion4/1
  Shift Arithmetic1/1 -> Bitwise Operator1/2
  OUT_Z_L/1 -> I2C Master Read/Write4/2
  OUT_Z_H/1 -> I2C Master Read/Write5/2
  I2C Master Read/Write5/2 -> Data Type Conversion2/1
  Data Type Conversion2/1 -> Shift Arithmetic2/1
  I2C Master Read/Write4/2 -> Data Type Conversion5/1
  Shift Arithmetic2/1 -> Bitwise Operator2/2
  Bitwise Operator2/1 -> Data Type Conversion8/1
  Data Type Conversion3/1 -> Bitwise Operator/1
  Data Type Conversion4/1 -> Bitwise Operator1/1
  Data Type Conversion5/1 -> Bitwise Operator2/1
  Bitwise Operator1/1 -> Data Type Conversion7/1
  Data Type Conversion6/1 -> OUT_X/1
  Data Type Conversion7/1 -> OUT_Y/1
  Data Type Conversion8/1 -> OUT_Z/1
  OUT_TEMP/1 -> I2C Master Read/Write6/2
  I2C Master Read/Write6/2 -> OUT_T/1
  SlvAddr/1 -> I2C Master Read/Write/1, I2C Master Read/Write1/1, I2C Master Read/Write2/1, I2C Master Read/Write3/1, I2C Master Read/Write4/1, I2C Master Read/Write5/1, I2C Master Read/Write6/1
  I2C Master Read/Write/1 -> Terminator/1
  I2C Master Read/Write1/1 -> Terminator1/1
  I2C Master Read/Write2/1 -> Terminator2/1
  I2C Master Read/Write3/1 -> Terminator3/1
  I2C Master Read/Write4/1 -> Terminator4/1
  I2C Master Read/Write5/1 -> Terminator5/1
  I2C Master Read/Write6/1 -> Terminator6/1

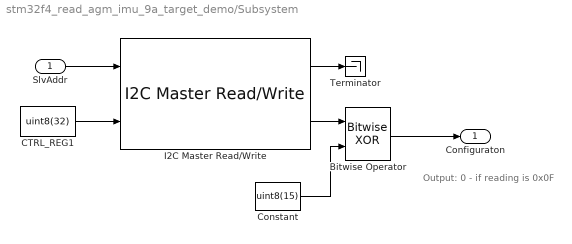
== system stm32f4_read_agm_imu_9a_target_demo/Subsystem ==
  note: Output:
      | 0 - if reading is 0x0F
  SlvAddr : Inport  OutDataType=fixdt(1, 16)  OutScaling=2^0
  Bitwise Operator : simulink/Logic and Bit Operations/Bitwise Operator  logicop=XOR  UseBitMask=off  NumInputPorts=2  BitMask=bin2dec('11011001')  BitMaskRealWorld=Stored Integer
  CTRL_REG1 : Constant  Value=uint8(32)  OutDataType=fixdt(1, 16)  OutScaling=2^0
  Constant : Constant  Value=uint8(15)  OutDataType=fixdt(1, 16)  OutScaling=2^0
  I2C Master Read/Write : stm32f4_i2c_lib/I2C Master Read//Write  configuration=Transaction  module=1  lastmodule=3  transfer=Blocking  dutycycle=TLow/THigh = 2  clkspeed=400  timeout=25  writecount=1  readcount=1  sdapin=C9  sclpin=A8  waitwritetime=0  forcestop=off  inputtypearray=[2 3 3]  outputtypearray=[2 3 3]  confstr="[\"C\",\"9\",\"A\",\"8\",\"1\",\"1\",\"6\",\"0\",\"I2C_DutyCycle_2\",\"0\",\"off\"]"  sampletime=-1  sampletimestr=0.01  blockid=SubsystemI2CMasterReadWrite
  Terminator : Terminator
  Configuraton : Outport  OutDataType=fixdt(1, 16)  OutScaling=2^0
  wires:
  I2C Master Read/Write/2 -> Bitwise Operator/1
  Bitwise Operator/1 -> Configuraton/1
  Constant/1 -> Bitwise Operator/2
  SlvAddr/1 -> I2C Master Read/Write/1
  CTRL_REG1/1 -> I2C Master Read/Write/2
  I2C Master Read/Write/1 -> Terminator/1

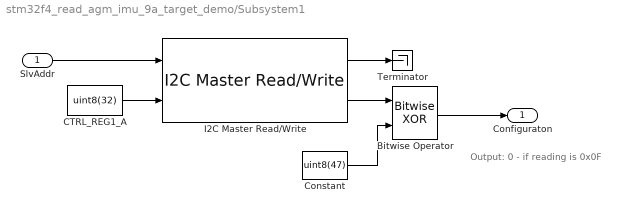
== system stm32f4_read_agm_imu_9a_target_demo/Subsystem1 ==
  note: Output:
      | 0 - if reading is 0x0F
  SlvAddr : Inport  OutDataType=fixdt(1, 16)  OutScaling=2^0
  Bitwise Operator : simulink/Logic and Bit Operations/Bitwise Operator  logicop=XOR  UseBitMask=off  NumInputPorts=2  BitMask=bin2dec('11011001')  BitMaskRealWorld=Stored Integer
  CTRL_REG1_A : Constant  Value=uint8(32)  OutDataType=fixdt(1, 16)  OutScaling=2^0
  Constant : Constant  Value=uint8(47)  OutDataType=fixdt(1, 16)  OutScaling=2^0
  I2C Master Read/Write : stm32f4_i2c_lib/I2C Master Read//Write  configuration=Transaction  module=1  lastmodule=3  transfer=Blocking  dutycycle=TLow/THigh = 2  clkspeed=400  timeout=25  writecount=1  readcount=1  sdapin=C9  sclpin=A8  waitwritetime=0  forcestop=off  inputtypearray=[2 3 3]  outputtypearray=[2 3 3]  confstr="[\"C\",\"9\",\"A\",\"8\",\"1\",\"1\",\"6\",\"0\",\"I2C_DutyCycle_2\",\"0\",\"off\"]"  sampletime=-1  sampletimestr=0.01  blockid=Subsystem1I2CMasterReadWrite
  Terminator : Terminator
  Configuraton : Outport  OutDataType=fixdt(1, 16)  OutScaling=2^0
  wires:
  Constant/1 -> Bitwise Operator/2
  Bitwise Operator/1 -> Configuraton/1
  I2C Master Read/Write/2 -> Bitwise Operator/1
  CTRL_REG1_A/1 -> I2C Master Read/Write/2
  SlvAddr/1 -> I2C Master Read/Write/1
  I2C Master Read/Write/1 -> Terminator/1

== system stm32f4_read_agm_imu_9a_target_demo/Subsystem2 ==
  note: Output:
      | 0 - if reading is 0x0F
  SlvAddr : Inport  OutDataType=fixdt(1, 16)  OutScaling=2^0
  Bitwise Operator : simulink/Logic and Bit Operations/Bitwise Operator  logicop=XOR  UseBitMask=off  NumInputPorts=2  BitMask=bin2dec('11011001')  BitMaskRealWorld=Stored Integer
  CTRL_REG1_M : Constant  Value=uint8(0)  OutDataType=fixdt(1, 16)  OutScaling=2^0
  Constant : Constant  Value=uint8(24)  OutDataType=fixdt(1, 16)  OutScaling=2^0
  I2C Master Read/Write : stm32f4_i2c_lib/I2C Master Read//Write  configuration=Transaction  module=1  lastmodule=3  transfer=Blocking  dutycycle=TLow/THigh = 2  clkspeed=400  timeout=25  writecount=1  readcount=1  sdapin=C9  sclpin=A8  waitwritetime=0  forcestop=off  inputtypearray=[2 3 3]  outputtypearray=[2 3 3]  confstr="[\"C\",\"9\",\"A\",\"8\",\"1\",\"1\",\"6\",\"0\",\"I2C_DutyCycle_2\",\"0\",\"off\"]"  sampletime=-1  sampletimestr=0.01  blockid=Subsystem2I2CMasterReadWrite
  Terminator : Terminator
  Configuraton : Outport  OutDataType=fixdt(1, 16)  OutScaling=2^0
  wires:
  I2C Master Read/Write/2 -> Bitwise Operator/1
  Bitwise Operator/1 -> Configuraton/1
  Constant/1 -> Bitwise Operator/2
  CTRL_REG1_M/1 -> I2C Master Read/Write/2
  SlvAddr/1 -> I2C Master Read/Write/1
  I2C Master Read/Write/1 -> Terminator/1

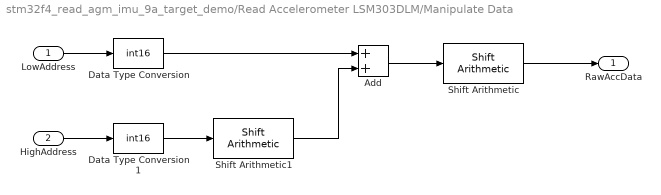
== system stm32f4_read_agm_imu_9a_target_demo/Read Accelerometer LSM303DLM/Manipulate Data ==
  LowAddress : Inport  OutDataType=fixdt(1, 16)  OutScaling=2^0
  HighAddress : Inport  Port=2  OutDataType=fixdt(1, 16)  OutScaling=2^0
  Add : Sum  OutDataType=fixdt(1, 16)  OutScaling=2^-10
  Data Type Conversion : DataTypeConversion  OutDataTypeMode=int16  OutDataType=fixdt(1, 16)  OutScaling=2^0  OutDataTypeStr=int16
  Data Type Conversion1 : DataTypeConversion  OutDataTypeMode=int16  OutDataType=fixdt(1, 16)  OutScaling=2^0  OutDataTypeStr=int16
  Shift Arithmetic : simulink/Logic and Bit Operations/Shift Arithmetic  SystemSampleTime=-1  nBitShiftRight=4  nBinPtShiftRight=0
  Shift Arithmetic1 : simulink/Logic and Bit Operations/Shift Arithmetic  SystemSampleTime=-1  nBitShiftRight=-8  nBinPtShiftRight=0
  RawAccData : Outport  OutDataType=fixdt(1, 16)  OutScaling=2^0
  wires:
  LowAddress/1 -> Data Type Conversion/1
  HighAddress/1 -> Data Type Conversion1/1
  Data Type Conversion/1 -> Add/1
  Data Type Conversion1/1 -> Shift Arithmetic1/1
  Shift Arithmetic1/1 -> Add/2
  Add/1 -> Shift Arithmetic/1
  Shift Arithmetic/1 -> RawAccData/1

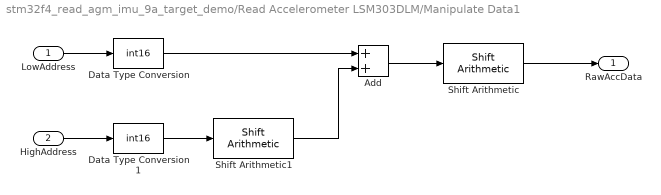
== system stm32f4_read_agm_imu_9a_target_demo/Read Accelerometer LSM303DLM/Manipulate Data1 ==
  LowAddress : Inport  OutDataType=fixdt(1, 16)  OutScaling=2^0
  HighAddress : Inport  Port=2  OutDataType=fixdt(1, 16)  OutScaling=2^0
  Add : Sum  OutDataType=fixdt(1, 16)  OutScaling=2^-10
  Data Type Conversion : DataTypeConversion  OutDataTypeMode=int16  OutDataType=fixdt(1, 16)  OutScaling=2^0  OutDataTypeStr=int16
  Data Type Conversion1 : DataTypeConversion  OutDataTypeMode=int16  OutDataType=fixdt(1, 16)  OutScaling=2^0  OutDataTypeStr=int16
  Shift Arithmetic : simulink/Logic and Bit Operations/Shift Arithmetic  SystemSampleTime=-1  nBitShiftRight=4  nBinPtShiftRight=0
  Shift Arithmetic1 : simulink/Logic and Bit Operations/Shift Arithmetic  SystemSampleTime=-1  nBitShiftRight=-8  nBinPtShiftRight=0
  RawAccData : Outport  OutDataType=fixdt(1, 16)  OutScaling=2^0
  wires:
  Shift Arithmetic/1 -> RawAccData/1
  Add/1 -> Shift Arithmetic/1
  Shift Arithmetic1/1 -> Add/2
  Data Type Conversion1/1 -> Shift Arithmetic1/1
  Data Type Conversion/1 -> Add/1
  HighAddress/1 -> Data Type Conversion1/1
  LowAddress/1 -> Data Type Conversion/1

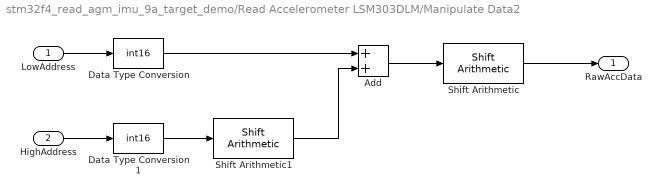
== system stm32f4_read_agm_imu_9a_target_demo/Read Accelerometer LSM303DLM/Manipulate Data2 ==
  LowAddress : Inport  OutDataType=fixdt(1, 16)  OutScaling=2^0
  HighAddress : Inport  Port=2  OutDataType=fixdt(1, 16)  OutScaling=2^0
  Add : Sum  OutDataType=fixdt(1, 16)  OutScaling=2^-10
  Data Type Conversion : DataTypeConversion  OutDataTypeMode=int16  OutDataType=fixdt(1, 16)  OutScaling=2^0  OutDataTypeStr=int16
  Data Type Conversion1 : DataTypeConversion  OutDataTypeMode=int16  OutDataType=fixdt(1, 16)  OutScaling=2^0  OutDataTypeStr=int16
  Shift Arithmetic : simulink/Logic and Bit Operations/Shift Arithmetic  SystemSampleTime=-1  nBitShiftRight=4  nBinPtShiftRight=0
  Shift Arithmetic1 : simulink/Logic and Bit Operations/Shift Arithmetic  SystemSampleTime=-1  nBitShiftRight=-8  nBinPtShiftRight=0
  RawAccData : Outport  OutDataType=fixdt(1, 16)  OutScaling=2^0
  wires:
  LowAddress/1 -> Data Type Conversion/1
  HighAddress/1 -> Data Type Conversion1/1
  Data Type Conversion/1 -> Add/1
  Data Type Conversion1/1 -> Shift Arithmetic1/1
  Shift Arithmetic1/1 -> Add/2
  Add/1 -> Shift Arithmetic/1
  Shift Arithmetic/1 -> RawAccData/1

== system stm32f4_read_agm_imu_9a_target_demo/Read Magnetometer LSM303DLM/Manipulate Data1 ==
  HighAddress : Inport  OutDataType=fixdt(1, 16)  OutScaling=2^0
  LowAddress : Inport  Port=2  OutDataType=fixdt(1, 16)  OutScaling=2^0
  Bitwise Operator : simulink/Logic and Bit Operations/Bitwise Operator  logicop=OR  UseBitMask=off  NumInputPorts=2  BitMask=bin2dec('11011001')  BitMaskRealWorld=Stored Integer
  Data Type Conversion : DataTypeConversion  OutDataTypeMode=int16  OutDataType=fixdt(1, 16)  OutScaling=2^0  OutDataTypeStr=int16
  Data Type Conversion1 : DataTypeConversion  OutDataTypeMode=int16  OutDataType=fixdt(1, 16)  OutScaling=2^0  OutDataTypeStr=int16
  Shift Arithmetic2 : simulink/Logic and Bit Operations/Shift Arithmetic  SystemSampleTime=-1  nBitShiftRight=-8  nBinPtShiftRight=0
  RawMagData : Outport  OutDataType=fixdt(1, 16)  OutScaling=2^0
  wires:
  Shift Arithmetic2/1 -> Bitwise Operator/1
  HighAddress/1 -> Data Type Conversion/1
  LowAddress/1 -> Data Type Conversion1/1
  Data Type Conversion/1 -> Shift Arithmetic2/1
  Data Type Conversion1/1 -> Bitwise Operator/2
  Bitwise Operator/1 -> RawMagData/1

== system stm32f4_read_agm_imu_9a_target_demo/Read Magnetometer LSM303DLM/Manipulate Data2 ==
  HighAddress : Inport  OutDataType=fixdt(1, 16)  OutScaling=2^0
  LowAddress : Inport  Port=2  OutDataType=fixdt(1, 16)  OutScaling=2^0
  Bitwise Operator : simulink/Logic and Bit Operations/Bitwise Operator  logicop=OR  UseBitMask=off  NumInputPorts=2  BitMask=bin2dec('11011001')  BitMaskRealWorld=Stored Integer
  Data Type Conversion : DataTypeConversion  OutDataTypeMode=int16  OutDataType=fixdt(1, 16)  OutScaling=2^0  OutDataTypeStr=int16
  Data Type Conversion1 : DataTypeConversion  OutDataTypeMode=int16  OutDataType=fixdt(1, 16)  OutScaling=2^0  OutDataTypeStr=int16
  Shift Arithmetic2 : simulink/Logic and Bit Operations/Shift Arithmetic  SystemSampleTime=-1  nBitShiftRight=-8  nBinPtShiftRight=0
  RawMagData : Outport  OutDataType=fixdt(1, 16)  OutScaling=2^0
  wires:
  Bitwise Operator/1 -> RawMagData/1
  Data Type Conversion1/1 -> Bitwise Operator/2
  Data Type Conversion/1 -> Shift Arithmetic2/1
  LowAddress/1 -> Data Type Conversion1/1
  HighAddress/1 -> Data Type Conversion/1
  Shift Arithmetic2/1 -> Bitwise Operator/1

== system stm32f4_read_agm_imu_9a_target_demo/Read Magnetometer LSM303DLM/Manipulate Data5 ==
  HighAddress : Inport  OutDataType=fixdt(1, 16)  OutScaling=2^0
  LowAddress : Inport  Port=2  OutDataType=fixdt(1, 16)  OutScaling=2^0
  Bitwise Operator : simulink/Logic and Bit Operations/Bitwise Operator  logicop=OR  UseBitMask=off  NumInputPorts=2  BitMask=bin2dec('11011001')  BitMaskRealWorld=Stored Integer
  Data Type Conversion : DataTypeConversion  OutDataTypeMode=int16  OutDataType=fixdt(1, 16)  OutScaling=2^0  OutDataTypeStr=int16
  Data Type Conversion1 : DataTypeConversion  OutDataTypeMode=int16  OutDataType=fixdt(1, 16)  OutScaling=2^0  OutDataTypeStr=int16
  Shift Arithmetic2 : simulink/Logic and Bit Operations/Shift Arithmetic  SystemSampleTime=-1  nBitShiftRight=-8  nBinPtShiftRight=0
  RawMagData : Outport  OutDataType=fixdt(1, 16)  OutScaling=2^0
  wires:
  Bitwise Operator/1 -> RawMagData/1
  Data Type Conversion1/1 -> Bitwise Operator/2
  Data Type Conversion/1 -> Shift Arithmetic2/1
  LowAddress/1 -> Data Type Conversion1/1
  HighAddress/1 -> Data Type Conversion/1
  Shift Arithmetic2/1 -> Bitwise Operator/1
